simulink model "fm_a"  (R2023a)
settings: Solver=FixedStepAuto  StartTime=0.0  StopTime=0.1  FixedStep=0.0001  RelTol=1e-3
settings Model: Creator=pasha  LastModifiedBy=tanov

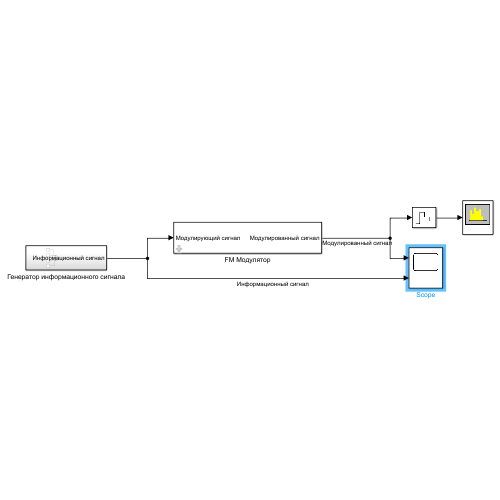
[thumbnail: Simulink's stored preview of the top-level diagram]
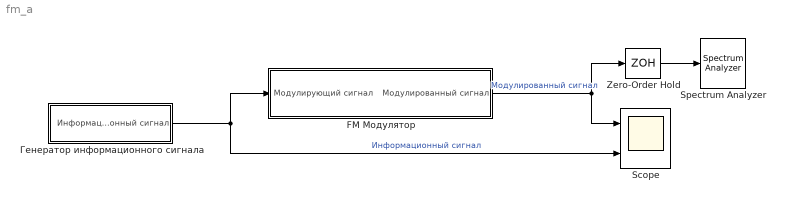
== system fm_a ==
  FM Модулятор : Subsystem  mask{f_c=300, w_d=250}
      mask prompts: f_c "Частота несущей"; w_d "Девиация Частоты"
  Scope : Scope  NumInputPorts=2
  Spectrum Analyzer : SpectrumAnalyzer  WindowPosition=[1.000000,49.000000,1600.000000,930.000000,]  ScopeFrameLocation=window  YLimits=[-58.76895037,31.63909406]
  Zero-Order Hold : ZeroOrderHold  SampleTime=1e-3
  Генератор информационного сигнала : Subsystem
  wires:
  Генератор информационного сигнала/1(Информационный сигнал) -> Scope/2, FM Модулятор/1(Модулирующий сигнал)  "Информационный сигнал"
  Zero-Order Hold/1 -> Spectrum Analyzer/1
  FM Модулятор/1(Модулированный сигнал) -> Scope/1, Zero-Order Hold/1  "Модулированный сигнал"

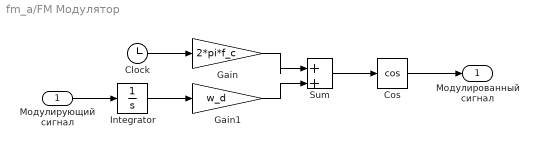
== system fm_a/FM Модулятор ==
  Модулирующий сигнал : Inport
  Clock : Clock
  Cos : Trigonometry  Operator=cos
  Gain : Gain  Gain=2*pi*f_c
  Gain1 : Gain  Gain=w_d
  Integrator : Integrator
  Sum : Sum  Inputs=|++
  Модулированный сигнал : Outport
  wires:
  Clock/1 -> Gain/1
  Sum/1 -> Cos/1
  Cos/1 -> Модулированный сигнал/1
  Модулирующий сигнал/1 -> Integrator/1
  Gain/1 -> Sum/1
  Integrator/1 -> Gain1/1
  Gain1/1 -> Sum/2

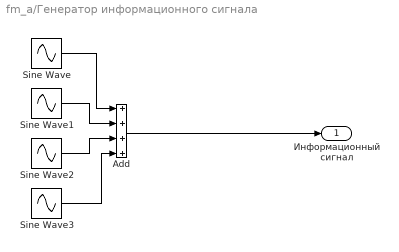
== system fm_a/Генератор информационного сигнала ==
  Add : Sum  Inputs=++++
  Sine Wave : Sin  Frequency=2*pi*40  SampleTime=0
  Sine Wave1 : Sin  Frequency=2*pi*60  SampleTime=0
  Sine Wave2 : Sin  Frequency=2*pi*80  SampleTime=0
  Sine Wave3 : Sin  Frequency=2*pi*100  SampleTime=0
  Информационный сигнал : Outport
  wires:
  Sine Wave/1 -> Add/1
  Sine Wave3/1 -> Add/4
  Sine Wave1/1 -> Add/2
  Sine Wave2/1 -> Add/3
  Add/1 -> Информационный сигнал/1
